simulink model "lqr_view"  (R2015a)
settings: Solver=ode45  StartTime=0.0  StopTime=10.0  RelTol=1e-3
values from neighbouring files (symbols this model uses):
  A = [0 1 ... (first row only)    [optimal_care.m]    (also in optimal_hamilton.m; optimal_servo.m = [ 0 1 0 0)
  B = [0 1]'    [optimal_care.m]    (also in optimal_hamilton.m; optimal_servo.m = [0 2 0 0]')
  K = -inv(R)*B'*P    [optimal_care.m]    (also in optimal_hamilton.m = -acker(A,B,lambda); optimal_servo.m = -inv(Re)*B'*P11)
  x0 = [1 0]'    [optimal_care.m]    (also in optimal_hamilton.m; optimal_servo.m = [0 0 0.25 0]')
settings Model: Creator=shohei  LastModifiedBy=shohei

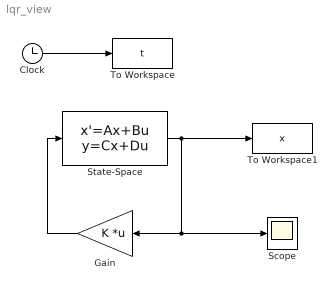
== system lqr_view ==
  Clock : Clock
  Gain : Gain  Gain=K  Multiplication=Matrix(K*u)
  Scope : Scope
  State-Space : StateSpace  A=A  B=B  C=eye(2)  D=zeros(2,1)  X0=x0
  To Workspace : ToWorkspace  VariableName=t  SaveFormat=Timeseries  SampleTime=-1
  To Workspace1 : ToWorkspace  VariableName=x  SaveFormat=Timeseries  SampleTime=-1
  wires:
  Clock/1 -> To Workspace/1
  State-Space/1 -> To Workspace1/1, Gain/1, Scope/1
  Gain/1 -> State-Space/1
